simulink model "missile_simulator"  (R2022b)
settings: Solver=VariableStepAuto  StartTime=0.0  StopTime=1000  RelTol=1e-3
settings Model: Creator=백창인  LastModifiedBy=백창인

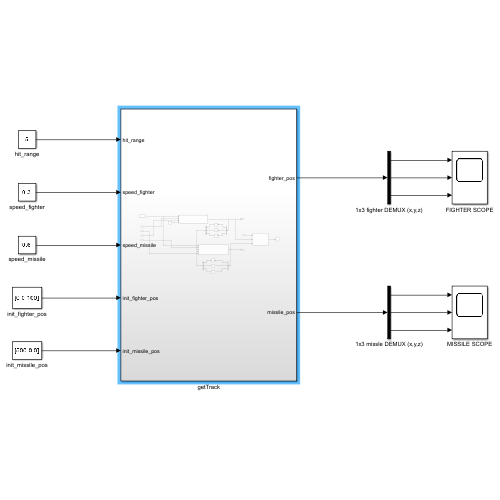
[thumbnail: Simulink's stored preview of the top-level diagram]
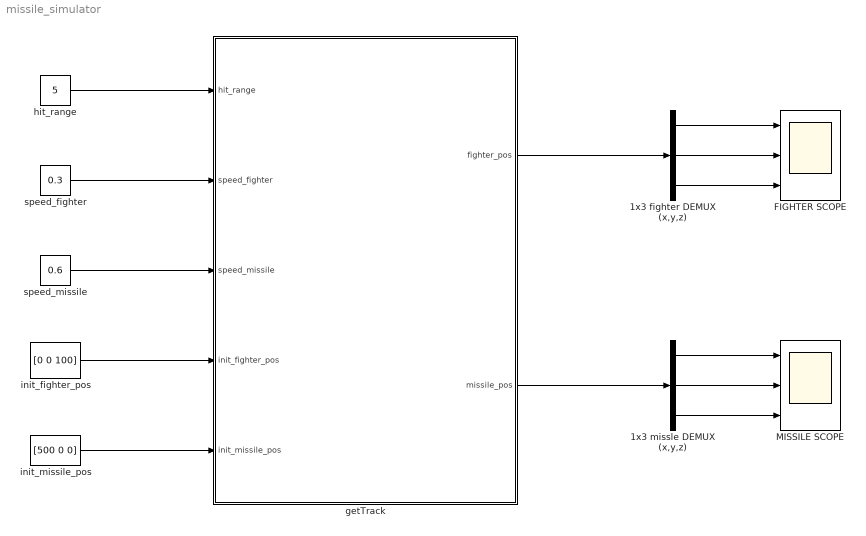
== system missile_simulator ==
  1x3 fighter DEMUX (x,y,z) : Demux  Outputs=3
  1x3 missle DEMUX (x,y,z) : Demux  Outputs=3
  FIGHTER SCOPE : Scope  NumInputPorts=3
  MISSILE SCOPE : Scope  NumInputPorts=3
  getTrack : Subsystem
  hit_range : Constant  Value=5
  init_fighter_pos : Constant  Value=[0 0 100]
  init_missile_pos : Constant  Value=[500 0 0]
  speed_fighter : Constant  Value=0.3
  speed_missile : Constant  Value=0.6
  wires:
  hit_range/1 -> getTrack/1(hit_range)
  speed_fighter/1 -> getTrack/2(speed_fighter)
  speed_missile/1 -> getTrack/3(speed_missile)
  init_fighter_pos/1 -> getTrack/4(init_fighter_pos)
  init_missile_pos/1 -> getTrack/5(init_missile_pos)
  getTrack/1(fighter_pos) -> 1x3 fighter DEMUX (x,y,z)/1
  1x3 fighter DEMUX (x,y,z)/1 -> FIGHTER SCOPE/1
  1x3 fighter DEMUX (x,y,z)/2 -> FIGHTER SCOPE/2
  1x3 fighter DEMUX (x,y,z)/3 -> FIGHTER SCOPE/3
  getTrack/2(missile_pos) -> 1x3 missle DEMUX (x,y,z)/1
  1x3 missle DEMUX (x,y,z)/1 -> MISSILE SCOPE/1
  1x3 missle DEMUX (x,y,z)/2 -> MISSILE SCOPE/2
  1x3 missle DEMUX (x,y,z)/3 -> MISSILE SCOPE/3

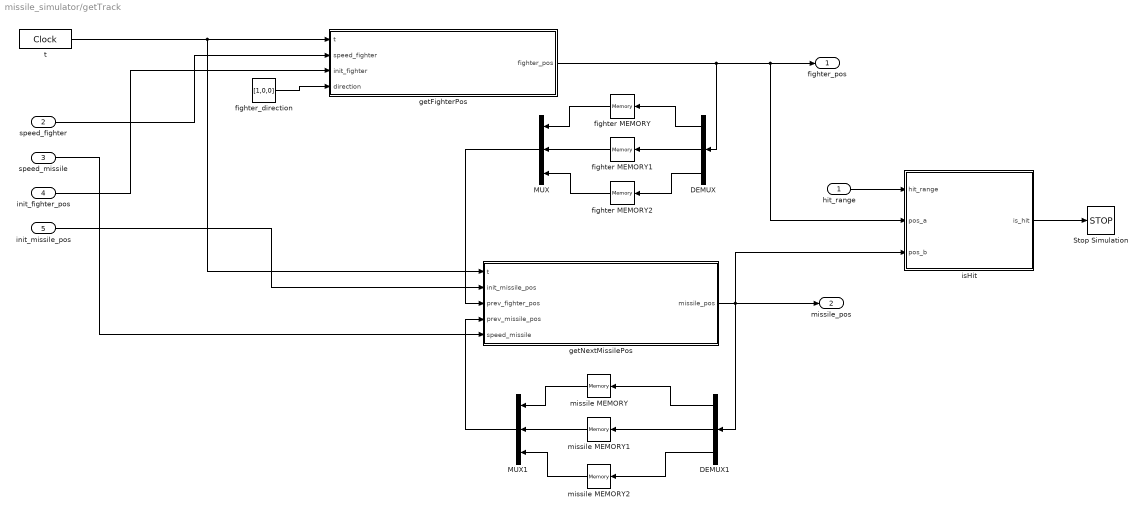
== system missile_simulator/getTrack ==
  hit_range : Inport
  speed_fighter : Inport  Port=2
  speed_missile : Inport  Port=3
  init_fighter_pos : Inport  Port=4
  init_missile_pos : Inport  Port=5
  DEMUX : Demux  Outputs=3
  DEMUX1 : Demux  Outputs=3
  MUX : Mux  Inputs=3
  MUX1 : Mux  Inputs=3
  Stop Simulation : Stop
  fighter MEMORY : Memory  LinearizeAsDelay=on
  fighter MEMORY1 : Memory  LinearizeAsDelay=on
  fighter MEMORY2 : Memory  LinearizeAsDelay=on
  fighter_direction : Constant  Value=[1,0,0]
  getFighterPos : MATLAB Function  TreatAsAtomicUnit=on
  getNextMissilePos : MATLAB Function  TreatAsAtomicUnit=on
  isHit : MATLAB Function  TreatAsAtomicUnit=on
  missile MEMORY : Memory  LinearizeAsDelay=on
  missile MEMORY1 : Memory  LinearizeAsDelay=on
  missile MEMORY2 : Memory  LinearizeAsDelay=on
  t : DigitalClock
  fighter_pos : Outport
  missile_pos : Outport  Port=2
  wires:
  t/1 -> getNextMissilePos/1(t), getFighterPos/1(t)
  getFighterPos/1(fighter_pos) -> DEMUX/1, isHit/2(pos_a), fighter_pos/1
  speed_fighter/1 -> getFighterPos/2(speed_fighter)
  init_fighter_pos/1 -> getFighterPos/3(init_fighter)
  fighter_direction/1 -> getFighterPos/4(direction)
  getNextMissilePos/1(missile_pos) -> isHit/3(pos_b), DEMUX1/1, missile_pos/1
  init_missile_pos/1 -> getNextMissilePos/2(init_missile_pos)
  speed_missile/1 -> getNextMissilePos/5(speed_missile)
  MUX1/1 -> getNextMissilePos/4(prev_missile_pos)
  MUX/1 -> getNextMissilePos/3(prev_fighter_pos)
  DEMUX/2 -> fighter MEMORY1/1
  DEMUX/1 -> fighter MEMORY/1
  DEMUX/3 -> fighter MEMORY2/1
  fighter MEMORY/1 -> MUX/1
  fighter MEMORY1/1 -> MUX/2
  fighter MEMORY2/1 -> MUX/3
  DEMUX1/1 -> missile MEMORY/1
  DEMUX1/2 -> missile MEMORY1/1
  DEMUX1/3 -> missile MEMORY2/1
  missile MEMORY1/1 -> MUX1/2
  missile MEMORY/1 -> MUX1/1
  missile MEMORY2/1 -> MUX1/3
  isHit/1(is_hit) -> Stop Simulation/1
  hit_range/1 -> isHit/1(hit_range)

== matlab function missile_simulator/getTrack/isHit ==
  data: hit_range input; is_hit output; pos_a input; pos_b input
function is_hit = isHit(hit_range, pos_a, pos_b)
    is_hit = 0;
    distance = norm(pos_a(end, :) - pos_b(end, :));

    if (distance <= hit_range)
        is_hit = 1;
    end
end

== matlab function missile_simulator/getTrack/getFighterPos ==
  data: t input; fighter_pos output; speed_fighter input; init_fighter input; direction input
function fighter_pos = getFighterPos(t,speed_fighter,init_fighter,direction)
    position = init_fighter + (t-1)*direction*speed_fighter; %전투기의 위치를 속도와 시간에 따라 재설정
fighter_pos = position;
end

== matlab function missile_simulator/getTrack/getNextMissilePos ==
  data: t input; init_missile_pos input; prev_fighter_pos input; prev_missile_pos input; missile_pos output; speed_missile input
function missile_pos = getNextMissilePos(t, init_missile_pos, prev_fighter_pos, prev_missile_pos, speed_missile)
% 방향벡터에 미사일 속도를 적용
if (t==1) %초기값
    missile_pos = init_missile_pos;
else
    direction = (prev_fighter_pos - prev_missile_pos); %미사일 방향벡터
    unit_direction = (direction)/norm(direction);
    missile_pos = prev_missile_pos + speed_missile * unit_direction;
end

end
